simulink model "PenduloInvertidoTorque"  (R2025a)
settings: Solver=ode45  StartTime=0.0  StopTime=10.0  RelTol=1e-3
libraries: fuzblock x1
settings Model: Creator=Lenovo  LastModifiedBy=Cubo3

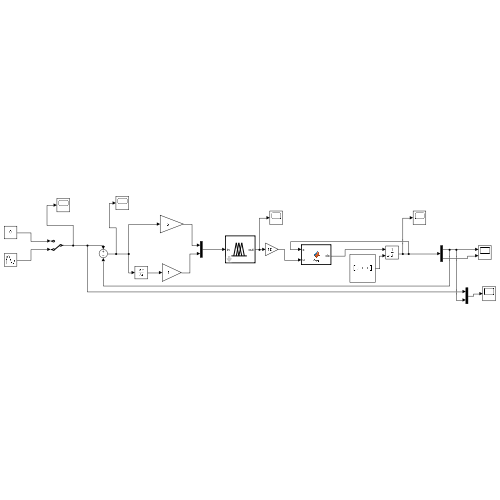
[thumbnail: Simulink's stored preview of the top-level diagram]
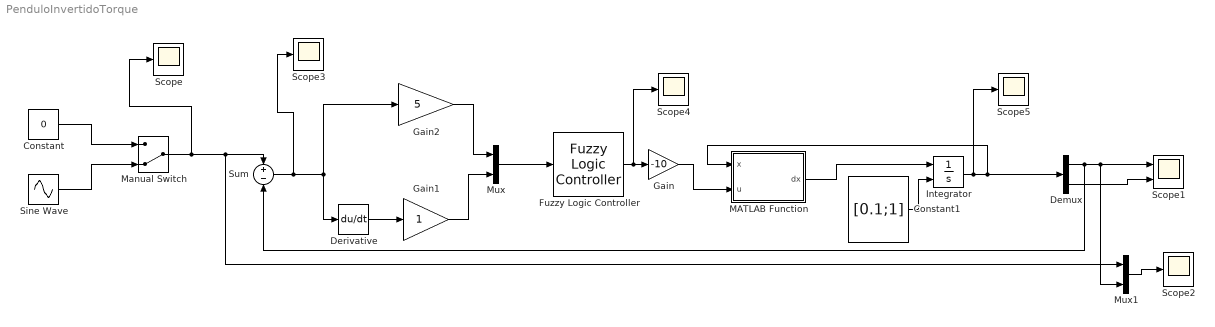
== system PenduloInvertidoTorque ==
  Constant : Constant  Value=0
  Constant1 : Constant  Value=[0.1;1]
  Demux : Demux  Outputs=2
  Derivative : Derivative
  Fuzzy Logic Controller : fuzblock/Fuzzy Logic  Controller  FIS='fuzzy_final'  OutputSampleNumber=101  DataType=double  UseLookupTable=off  NumBreakpoints=10  FuzzifiedInputs=off  RuleFiringStrengths=off  RuleOutputs=off  AggregatedOutputs=off  SimulateUsing=Interpreted execution  OutOfRangeInputValueMessage=warning  NoRuleFiredMessage=warning  EmptyOutputFuzzySetMessage=warning
  Gain : Gain  Gain=-10
  Gain1 : Gain
  Gain2 : Gain  Gain=5
  Integrator : Integrator  InitialConditionSource=external
  MATLAB Function : MATLAB Function  TreatAsAtomicUnit=on
  Manual Switch : ManualSwitch  CurrentSetting=0
  Mux : Mux  Inputs=2
  Mux1 : Mux  Inputs=2
  Scope{,2..5} (5 alike) : Scope
      Scope settings: ActiveDisplayYMinimum=-1  ActiveDisplayYMaximum=1
      Scope2 settings: ActiveDisplayYMinimum=-0.31999772930871817  ActiveDisplayYMaximum=0.36329385797761971  DataLoggingVariableName=ScopeData2
      Scope3 settings: ActiveDisplayYMinimum=-1  ActiveDisplayYMaximum=1  DataLoggingVariableName=ScopeData3
      Scope4 settings: ActiveDisplayYMinimum=-1  ActiveDisplayYMaximum=1  DataLoggingVariableName=ScopeData4
      Scope5 settings: ActiveDisplayYMinimum=-1  ActiveDisplayYMaximum=1  DataLoggingVariableName=ScopeData5
  Scope1 : Scope  NumInputPorts=2
      settings: ActiveDisplayYMinimum=-1.3058718130667684  ActiveDisplayYMaximum=1.2633229868655125
  Sine Wave : Sin  Amplitude=.25  Frequency=4  SampleTime=0
  Sum : Sum  Inputs=+-
  wires:
  Gain/1 -> MATLAB Function/2(u)
  Integrator/1 -> Scope5/1, Demux/1, MATLAB Function/1(x)
  MATLAB Function/1(dx) -> Integrator/1
  Constant1/1 -> Integrator/2
  Demux/1 -> Sum/2, Mux1/2, Scope1/1
  Demux/2 -> Scope1/2
  Fuzzy Logic Controller/1 -> Scope4/1, Gain/1
  Sine Wave/1 -> Manual Switch/2
  Constant/1 -> Manual Switch/1
  Mux/1 -> Fuzzy Logic Controller/1
  Gain1/1 -> Mux/2
  Gain2/1 -> Mux/1
  Manual Switch/1 -> Scope/1, Mux1/1, Sum/1
  Derivative/1 -> Gain1/1
  Mux1/1 -> Scope2/1
  Sum/1 -> Scope3/1, Derivative/1, Gain2/1

== matlab function PenduloInvertidoTorque/MATLAB Function ==
  data: x input; dx output; u input
function dx  = fcn(x,u)

l=1; m=1; g=9.81; b=0.5; I=m*l^2;
x1=x(1);
x2=x(2);
dx1=x2;
dx2=g/l*sin(x1)-b*l/I*x2+u/I;
dx = [dx1;dx2];
